simulink model "cosmic_ray_system_top"  (R2019a)
settings: Solver=VariableStepAuto  StartTime=0.0  StopTime=10.0  RelTol=1e-3
libraries: xbsIndex_r4 x3434, casper_library_misc x148, xps_library x3, casper_library_delays x1
(part 8 of 27)

== system cosmic_ray_system_top/Subsystem/wait_between_packets ==
  sim_1 : Inport
  convert1_1 : DataTypeConversion  OutDataTypeStr=fixdt('ufix32_En0')  LockScale=on
  convert2_1 : DataTypeConversion  OutDataTypeStr=fixdt('ufix32_En0')  ConvertRealWorld=Stored Integer (SI)  LockScale=on
  cosmic_ray_system_top_Subsystem_wait_between_packets_user_data_out : xbsIndex_r4/Gateway In  gui_display_data_type=Fixed-point  arith_type=Unsigned  n_bits=32  bin_pt=0  preci_type=Single  exp_width=8  frac_width=24  rows=1  columns=1  quantization="Round  (unbiased: +/- Inf)"  overflow=Saturate  period=1  UseAsADC=off  ADCChannel='1'  interface=None  automatic_assignment=on  address_offset=hex2dec('00')  intf_name=''  intf_description=''  default_value=0  timing_constraint=None  locs_specified=off  LOCs={}  io_standard={}  inherit_from_input=off  hdl_port=on  dbl_ovrd=off  block_type=gatewayin
  gain_1 : Gain
  io_delay : xbsIndex_r4/Delay  rst=off  infoeditControl=Selection of Reset will increase slice count due to use of real FFs and instead of SRLs  en=off  latency=0  reg_retiming=on  dbl_ovrd=off  block_type=delay
  reint1 : xbsIndex_r4/Reinterpret  force_arith_type=on  arith_type=Unsigned  force_bin_pt=on  bin_pt=0  block_type=reinterpret
  slice_reg : xbsIndex_r4/Slice  nbits=32  boolean_output=off  mode=Lower Bit Location + Width  bit1=0  base1=MSB of Input  bit0=0  base0=LSB of Input  dbl_ovrd=off  block_type=slice
  in_reg : Outport
  wires:
  cosmic_ray_system_top_Subsystem_wait_between_packets_user_data_out/1 -> io_delay/1
  sim_1/1 -> convert1_1/1
  convert1_1/1 -> convert2_1/1
  convert2_1/1 -> gain_1/1
  gain_1/1 -> cosmic_ray_system_top_Subsystem_wait_between_packets_user_data_out/1
  io_delay/1 -> slice_reg/1
  slice_reg/1 -> reint1/1
  reint1/1 -> in_reg/1

== system cosmic_ray_system_top/Subsystem/buffer_and_packetizer/bus_create ==
  in1 : Inport
  in2 : Inport  Port=2
  in3 : Inport  Port=3
  concatenate : xbsIndex_r4/Concat  num_inputs=3  dbl_ovrd=off  block_type=concat
  reinterpret1 : xbsIndex_r4/Reinterpret  force_arith_type=on  arith_type=Unsigned  force_bin_pt=on  bin_pt=0  block_type=reinterpret
      settings: infoedit="Changes signal type without altering the binary representation.   You can changed the signal between signed and unsigned, and relocate the binary point.<br><br>Hardware notes: In hardware this block costs nothing.<br><br>Example:  Suppose the input is 6 bits wide, signed, with 2 fractional bits, and the output is forced to unsigned with 0 fractional bits.  Then an input of -2.0 (1110.00 in binary 2's complement) becomes an output of 56 (111000 in binary)."
  reinterpret2 : xbsIndex_r4/Reinterpret  force_arith_type=on  arith_type=Unsigned  force_bin_pt=on  bin_pt=0  block_type=reinterpret
      settings: infoedit="Changes signal type without altering the binary representation.   You can changed the signal between signed and unsigned, and relocate the binary point.<br><br>Hardware notes: In hardware this block costs nothing.<br><br>Example:  Suppose the input is 6 bits wide, signed, with 2 fractional bits, and the output is forced to unsigned with 0 fractional bits.  Then an input of -2.0 (1110.00 in binary 2's complement) becomes an output of 56 (111000 in binary)."
  reinterpret3 : xbsIndex_r4/Reinterpret  force_arith_type=on  arith_type=Unsigned  force_bin_pt=on  bin_pt=0  block_type=reinterpret
  bus_out : Outport
  wires:
  concatenate/1 -> bus_out/1
  in1/1 -> reinterpret1/1
  reinterpret1/1 -> concatenate/1
  in2/1 -> reinterpret2/1
  reinterpret2/1 -> concatenate/2
  in3/1 -> reinterpret3/1
  reinterpret3/1 -> concatenate/3

== system cosmic_ray_system_top/Subsystem/buffer_and_packetizer/bus_create1 ==
  in1 : Inport
  in2 : Inport  Port=2
  in3 : Inport  Port=3
  concatenate : xbsIndex_r4/Concat  num_inputs=3  dbl_ovrd=off  block_type=concat
  reinterpret1 : xbsIndex_r4/Reinterpret  force_arith_type=on  arith_type=Unsigned  force_bin_pt=on  bin_pt=0  block_type=reinterpret
      settings: infoedit="Changes signal type without altering the binary representation.   You can changed the signal between signed and unsigned, and relocate the binary point.<br><br>Hardware notes: In hardware this block costs nothing.<br><br>Example:  Suppose the input is 6 bits wide, signed, with 2 fractional bits, and the output is forced to unsigned with 0 fractional bits.  Then an input of -2.0 (1110.00 in binary 2's complement) becomes an output of 56 (111000 in binary)."
  reinterpret2 : xbsIndex_r4/Reinterpret  force_arith_type=on  arith_type=Unsigned  force_bin_pt=on  bin_pt=0  block_type=reinterpret
      settings: infoedit="Changes signal type without altering the binary representation.   You can changed the signal between signed and unsigned, and relocate the binary point.<br><br>Hardware notes: In hardware this block costs nothing.<br><br>Example:  Suppose the input is 6 bits wide, signed, with 2 fractional bits, and the output is forced to unsigned with 0 fractional bits.  Then an input of -2.0 (1110.00 in binary 2's complement) becomes an output of 56 (111000 in binary)."
  reinterpret3 : xbsIndex_r4/Reinterpret  force_arith_type=on  arith_type=Unsigned  force_bin_pt=on  bin_pt=0  block_type=reinterpret
  bus_out : Outport
  wires:
  reinterpret3/1 -> concatenate/3
  in3/1 -> reinterpret3/1
  reinterpret2/1 -> concatenate/2
  in2/1 -> reinterpret2/1
  reinterpret1/1 -> concatenate/1
  in1/1 -> reinterpret1/1
  concatenate/1 -> bus_out/1

== system cosmic_ray_system_top/Subsystem/buffer_and_packetizer/bus_create2 ==
  in1 : Inport
  in2 : Inport  Port=2
  in3 : Inport  Port=3
  concatenate : xbsIndex_r4/Concat  num_inputs=3  dbl_ovrd=off  block_type=concat
  reinterpret1 : xbsIndex_r4/Reinterpret  force_arith_type=on  arith_type=Unsigned  force_bin_pt=on  bin_pt=0  block_type=reinterpret
      settings: infoedit="Changes signal type without altering the binary representation.   You can changed the signal between signed and unsigned, and relocate the binary point.<br><br>Hardware notes: In hardware this block costs nothing.<br><br>Example:  Suppose the input is 6 bits wide, signed, with 2 fractional bits, and the output is forced to unsigned with 0 fractional bits.  Then an input of -2.0 (1110.00 in binary 2's complement) becomes an output of 56 (111000 in binary)."
  reinterpret2 : xbsIndex_r4/Reinterpret  force_arith_type=on  arith_type=Unsigned  force_bin_pt=on  bin_pt=0  block_type=reinterpret
      settings: infoedit="Changes signal type without altering the binary representation.   You can changed the signal between signed and unsigned, and relocate the binary point.<br><br>Hardware notes: In hardware this block costs nothing.<br><br>Example:  Suppose the input is 6 bits wide, signed, with 2 fractional bits, and the output is forced to unsigned with 0 fractional bits.  Then an input of -2.0 (1110.00 in binary 2's complement) becomes an output of 56 (111000 in binary)."
  reinterpret3 : xbsIndex_r4/Reinterpret  force_arith_type=on  arith_type=Unsigned  force_bin_pt=on  bin_pt=0  block_type=reinterpret
  bus_out : Outport
  wires:
  concatenate/1 -> bus_out/1
  in1/1 -> reinterpret1/1
  reinterpret1/1 -> concatenate/1
  in2/1 -> reinterpret2/1
  reinterpret2/1 -> concatenate/2
  in3/1 -> reinterpret3/1
  reinterpret3/1 -> concatenate/3

== system cosmic_ray_system_top/Subsystem/buffer_and_packetizer/bus_create3 ==
  in1 : Inport
  in2 : Inport  Port=2
  in3 : Inport  Port=3
  concatenate : xbsIndex_r4/Concat  num_inputs=3  dbl_ovrd=off  block_type=concat
  reinterpret1 : xbsIndex_r4/Reinterpret  force_arith_type=on  arith_type=Unsigned  force_bin_pt=on  bin_pt=0  block_type=reinterpret
      settings: infoedit="Changes signal type without altering the binary representation.   You can changed the signal between signed and unsigned, and relocate the binary point.<br><br>Hardware notes: In hardware this block costs nothing.<br><br>Example:  Suppose the input is 6 bits wide, signed, with 2 fractional bits, and the output is forced to unsigned with 0 fractional bits.  Then an input of -2.0 (1110.00 in binary 2's complement) becomes an output of 56 (111000 in binary)."
  reinterpret2 : xbsIndex_r4/Reinterpret  force_arith_type=on  arith_type=Unsigned  force_bin_pt=on  bin_pt=0  block_type=reinterpret
      settings: infoedit="Changes signal type without altering the binary representation.   You can changed the signal between signed and unsigned, and relocate the binary point.<br><br>Hardware notes: In hardware this block costs nothing.<br><br>Example:  Suppose the input is 6 bits wide, signed, with 2 fractional bits, and the output is forced to unsigned with 0 fractional bits.  Then an input of -2.0 (1110.00 in binary 2's complement) becomes an output of 56 (111000 in binary)."
  reinterpret3 : xbsIndex_r4/Reinterpret  force_arith_type=on  arith_type=Unsigned  force_bin_pt=on  bin_pt=0  block_type=reinterpret
  bus_out : Outport
  wires:
  reinterpret3/1 -> concatenate/3
  in3/1 -> reinterpret3/1
  reinterpret2/1 -> concatenate/2
  in2/1 -> reinterpret2/1
  reinterpret1/1 -> concatenate/1
  in1/1 -> reinterpret1/1
  concatenate/1 -> bus_out/1

== system cosmic_ray_system_top/Subsystem/buffer_and_packetizer/bus_expand ==
  bus_in : Inport
  reinterpret{1..4} (4 alike) : xbsIndex_r4/Reinterpret  force_arith_type=on  arith_type=Unsigned  force_bin_pt=on  bin_pt=0  block_type=reinterpret
  slice1 : xbsIndex_r4/Slice  nbits=160  boolean_output=off  mode=Upper Bit Location + Width  bit1=-480  base1=MSB of Input  bit0=0  base0=LSB of Input  dbl_ovrd=off  block_type=slice
  slice2 : xbsIndex_r4/Slice  nbits=160  boolean_output=off  mode=Upper Bit Location + Width  bit1=-320  base1=MSB of Input  bit0=0  base0=LSB of Input  dbl_ovrd=off  block_type=slice
  slice3 : xbsIndex_r4/Slice  nbits=160  boolean_output=off  mode=Upper Bit Location + Width  bit1=-160  base1=MSB of Input  bit0=0  base0=LSB of Input  dbl_ovrd=off  block_type=slice
  slice4 : xbsIndex_r4/Slice  nbits=160  boolean_output=off  mode=Upper Bit Location + Width  bit1=0  base1=MSB of Input  bit0=0  base0=LSB of Input  dbl_ovrd=off  block_type=slice
  msb_out4 : Outport
  out3 : Outport  Port=2
  out2 : Outport  Port=3
  lsb_out1 : Outport  Port=4
  wires:
  bus_in/1 -> slice4/1, slice3/1, slice2/1, slice1/1
  slice4/1 -> reinterpret4/1
  reinterpret4/1 -> msb_out4/1
  slice3/1 -> reinterpret3/1
  reinterpret3/1 -> out3/1
  slice2/1 -> reinterpret2/1
  reinterpret2/1 -> out2/1
  slice1/1 -> reinterpret1/1
  reinterpret1/1 -> lsb_out1/1

== system cosmic_ray_system_top/Subsystem/buffer_and_packetizer/count-limited-counter ==
  en : Inport
  limit : Inport  Port=2
  Relational2 : xbsIndex_r4/Relational  mode=a>=b  op_type=Bool  en=off  latency=0  dbl_ovrd=off  block_type=relational
  word_counter1 : xbsIndex_r4/Counter  cnt_type=Free Running  cnt_to=257  operation=Up  start_count=0  cnt_by_val=1  arith_type=Unsigned  n_bits=32  bin_pt=0  load_pin=off  rst=on  en=on  explicit_period=on  period=1  use_behavioral_HDL=off  implementation=Fabric  dbl_ovrd=off  block_type=counter
  out : Outport
  wires:
  Relational2/1 -> word_counter1/1
  word_counter1/1 -> out/1, Relational2/1
  en/1 -> word_counter1/2
  limit/1 -> Relational2/2

== system cosmic_ray_system_top/Subsystem/buffer_and_packetizer/edge_detect11 ==
  in : Inport
  Delay : xbsIndex_r4/Delay  rst=off  infoeditControl=Selection of Reset will increase slice count due to use of real FFs and instead of SRLs  en=off  latency=1  reg_retiming=off  dbl_ovrd=off  block_type=delay
      settings: xl_area=[0, 0, 0, 0, 0, 0, 0]
  Inverter : xbsIndex_r4/Inverter  en=off  latency=0  dbl_ovrd=off  block_type=inv
      settings: xl_area=[0, 0, 0, 0, 0, 0, 0]
  edge_op : xbsIndex_r4/Logical  logical_function=AND  inputs=2  en=off  latency=0  precision=Full  arith_type=Unsigned  n_bits=8  bin_pt=2  align_bp=on  dbl_ovrd=off  block_type=logical
      settings: xl_area=[0, 0, 0, 0, 0, 0, 0]
  out : Outport
  wires:
  Delay/1 -> edge_op/2
  in/1 -> Delay/1, Inverter/1
  edge_op/1 -> out/1
  Inverter/1 -> edge_op/1

== system cosmic_ray_system_top/Subsystem/buffer_and_packetizer/edge_detect12 ==
  in : Inport
  Delay : xbsIndex_r4/Delay  rst=off  infoeditControl=Selection of Reset will increase slice count due to use of real FFs and instead of SRLs  en=off  latency=1  reg_retiming=off  dbl_ovrd=off  block_type=delay
      settings: xl_area=[0, 0, 0, 0, 0, 0, 0]
  Inverter : xbsIndex_r4/Inverter  en=off  latency=0  dbl_ovrd=off  block_type=inv
      settings: xl_area=[0, 0, 0, 0, 0, 0, 0]
  edge_op : xbsIndex_r4/Logical  logical_function=AND  inputs=2  en=off  latency=0  precision=Full  arith_type=Unsigned  n_bits=8  bin_pt=2  align_bp=on  dbl_ovrd=off  block_type=logical
      settings: xl_area=[0, 0, 0, 0, 0, 0, 0]
  out : Outport
  wires:
  Delay/1 -> edge_op/2
  in/1 -> Delay/1, Inverter/1
  edge_op/1 -> out/1
  Inverter/1 -> edge_op/1

== system cosmic_ray_system_top/Subsystem/buffer_and_packetizer/edge_detect13 ==
  in : Inport
  Delay : xbsIndex_r4/Delay  rst=off  infoeditControl=Selection of Reset will increase slice count due to use of real FFs and instead of SRLs  en=off  latency=1  reg_retiming=off  dbl_ovrd=off  block_type=delay
      settings: xl_area=[0, 0, 0, 0, 0, 0, 0]
  Inverter : xbsIndex_r4/Inverter  en=off  latency=0  dbl_ovrd=off  block_type=inv
      settings: xl_area=[0, 0, 0, 0, 0, 0, 0]
  edge_op : xbsIndex_r4/Logical  logical_function=AND  inputs=2  en=off  latency=0  precision=Full  arith_type=Unsigned  n_bits=8  bin_pt=2  align_bp=on  dbl_ovrd=off  block_type=logical
      settings: xl_area=[0, 0, 0, 0, 0, 0, 0]
  out : Outport
  wires:
  Inverter/1 -> edge_op/1
  edge_op/1 -> out/1
  in/1 -> Inverter/1, Delay/1
  Delay/1 -> edge_op/2

== system cosmic_ray_system_top/Subsystem/coincidence_trigger/bus_relational ==
  a : Inport
  b : Inport  Port=2
  misci : Inport  Port=3
  a_debus : Subsystem  AncestorBlock=casper_library_flow_control/bus_expand  mask(bus_expand){mode=divisions of arbitrary size, outputNum=1, outputWidth=[11  11  11  11  11  11  11  11  11  11  11  11  11  11  11  11  11  11  11  11  11  11  11  11  11  11  11  11  11  11  11  11  11  11  11  11  11  11  11  11  11  11  11  11  11  11  11  11  11  11  11  11  11  11  11  11  11  11  11  11  11  11  11  11], outputBinaryPt=[0  0  0  0  0  0  0  0  0  0  0  0  0  0  0  0  0  0  0  0  0  0  0  0  0  0  0  0  0  0  0  0  0  0  0  0  0  0  0  0  0  0  0  0  0  0  0  0  0  0  0  0  0  0  0  0  0  0  0  0  0  0  0  0], outputArithmeticType=[0  0  0  0  0  0  0  0  0  0  0  0  0  0  0  0  0  0  0  0  0  0  0  0  0  0  0  0  0  0  0  0  0  0  0  0  0  0  0  0  0  0  0  0  0  0  0  0  0  0  0  0  0  0  0  0  0  0  0  0  0  0  0  0], show_format=on, outputToWorkspace=off, variablePrefix=, outputToModelAsWell=on}
      mask prompts: outputNum "Number of outputs:"; outputWidth "Output width [msb ... lsb]:"; outputBinaryPt "Output binary point position [msb ... lsb]:"; outputArithmeticType "Output arithmetic type (ufix=0, fix=1, bool=2) [msb ... lsb]:"; show_format "Print format string?"; outputToWorkspace "Output to workspace?"; variablePrefix "Variable name prefix:"; outputToModelAsWell "Output to model as well?"
      mask help:
      | Expands a 'bus' made using a bus_create or Xilinx
      | concat block.
      | The input will be divided into the specified number
      | of outputs with the specified arithmetic types.
      | Divisions are made from most significant bit.
      mask init: same as cosmic_ray_system_top/Subsystem/buffer_and_packetizer/bus_expand
      settings: AttributesFormatString=64 outputs: uf11.0,uf11.0,uf11.0,uf11.0,uf11.0,uf11.0,uf11.0,uf11.0,uf11.0,uf11.0,uf11.0,uf11.0,uf11.0,uf11.0,uf11.0,uf11.0,uf11.0,uf11.0,uf11.0,uf11.0,uf11.0,uf11.0,uf11.0,uf11.0,uf11.0,uf11.0,uf11.0,uf11.0,uf11.0,uf11.0,uf11.0,uf11.0,uf11.0,uf11.0,uf11.0,uf11.0,uf11.0,uf11.0,uf11.0,uf11.0,uf11.0,uf11.0,uf11.0,uf11.0,uf11.0,uf11.0,uf11.0,uf11.0,uf11.0,uf11.0,uf11.0,uf11.0,uf11.0,uf11.0,uf11.0,uf11.0,uf11.0,uf11.0,uf11.0,uf11.0,uf11.0,uf11.0,uf11.0,uf11.0,
      mask TypeOptions mode: divisions of equal size | divisions of arbitrary size
      mask Callback mode: bus_expand_callback();
      mask Callback outputWidth: bus_expand_callback();
      mask Callback outputToWorkspace: bus_expand_callback();
  b_debus : Subsystem  AncestorBlock=casper_library_flow_control/bus_expand  mask(bus_expand){mode=divisions of arbitrary size, outputNum=1, outputWidth=[12], outputBinaryPt=[0], outputArithmeticType=[0], show_format=on, outputToWorkspace=off, variablePrefix=, outputToModelAsWell=on}
      mask prompts: outputNum "Number of outputs:"; outputWidth "Output width [msb ... lsb]:"; outputBinaryPt "Output binary point position [msb ... lsb]:"; outputArithmeticType "Output arithmetic type (ufix=0, fix=1, bool=2) [msb ... lsb]:"; show_format "Print format string?"; outputToWorkspace "Output to workspace?"; variablePrefix "Variable name prefix:"; outputToModelAsWell "Output to model as well?"
      mask help:
      | Expands a 'bus' made using a bus_create or Xilinx
      | concat block.
      | The input will be divided into the specified number
      | of outputs with the specified arithmetic types.
      | Divisions are made from most significant bit.
      mask init: same as cosmic_ray_system_top/Subsystem/buffer_and_packetizer/bus_expand
      settings: AttributesFormatString=1 outputs: uf12.0,
      mask TypeOptions mode: divisions of equal size | divisions of arbitrary size
      mask Callback mode: bus_expand_callback();
      mask Callback outputWidth: bus_expand_callback();
      mask Callback outputToWorkspace: bus_expand_callback();
  bussify : Subsystem  AncestorBlock=casper_library_flow_control/bus_create  mask(bus_create){inputNum=64}
      mask prompts: inputNum "Number of inputs:"
      mask init:
      | bus_create_init(gcb,...
      |     'inputNum', inputNum);
  dmisc : xbsIndex_r4/Delay  rst=off  infoeditControl=Selection of Reset will increase slice count due to use of real FFs and instead of SRLs  en=off  latency=1  reg_retiming=on  dbl_ovrd=off  block_type=delay
  relational{1..64} (64 alike) : xbsIndex_r4/Relational  mode=a>b  op_type=Bool  en=off  latency=1  dbl_ovrd=off  block_type=relational
  a>b : Outport
  misco : Outport  Port=2
  wires:
  a/1 -> a_debus/1(bus_in)
  b/1 -> b_debus/1(bus_in)
  a_debus/1(msb_out64) -> relational1/1
  b_debus/1(msb_lsb_out1) -> relational1/2, relational2/2, relational3/2, relational4/2, relational5/2, relational6/2, relational7/2, relational8/2, relational9/2, relational10/2, relational11/2, relational12/2, relational13/2, relational14/2, relational15/2, relational16/2, relational17/2, relational18/2, relational19/2, relational20/2, relational21/2, relational22/2, relational23/2, relational24/2, relational25/2, relational26/2, relational27/2, relational28/2, relational29/2, relational30/2, relational31/2, relational32/2, relational33/2, relational34/2, relational35/2, relational36/2, relational37/2, relational38/2, relational39/2, relational40/2, relational41/2, relational42/2, relational43/2, relational44/2, relational45/2, relational46/2, relational47/2, relational48/2, relational49/2, relational50/2, relational51/2, relational52/2, relational53/2, relational54/2, relational55/2, relational56/2, relational57/2, relational58/2, relational59/2, relational60/2, relational61/2, relational62/2, relational63/2, relational64/2
  a_debus/2(out63) -> relational2/1
  a_debus/3(out62) -> relational3/1
  a_debus/4(out61) -> relational4/1
  a_debus/5(out60) -> relational5/1
  a_debus/6(out59) -> relational6/1
  a_debus/7(out58) -> relational7/1
  a_debus/8(out57) -> relational8/1
  a_debus/9(out56) -> relational9/1
  a_debus/10(out55) -> relational10/1
  a_debus/11(out54) -> relational11/1
  a_debus/12(out53) -> relational12/1
  a_debus/13(out52) -> relational13/1
  a_debus/14(out51) -> relational14/1
  a_debus/15(out50) -> relational15/1
  a_debus/16(out49) -> relational16/1
  a_debus/17(out48) -> relational17/1
  a_debus/18(out47) -> relational18/1
  a_debus/19(out46) -> relational19/1
  a_debus/20(out45) -> relational20/1
  a_debus/21(out44) -> relational21/1
  a_debus/22(out43) -> relational22/1
  a_debus/23(out42) -> relational23/1
  a_debus/24(out41) -> relational24/1
  a_debus/25(out40) -> relational25/1
  a_debus/26(out39) -> relational26/1
  a_debus/27(out38) -> relational27/1
  a_debus/28(out37) -> relational28/1
  a_debus/29(out36) -> relational29/1
  a_debus/30(out35) -> relational30/1
  a_debus/31(out34) -> relational31/1
  a_debus/32(out33) -> relational32/1
  a_debus/33(out32) -> relational33/1
  a_debus/34(out31) -> relational34/1
  a_debus/35(out30) -> relational35/1
  a_debus/36(out29) -> relational36/1
  a_debus/37(out28) -> relational37/1
  a_debus/38(out27) -> relational38/1
  a_debus/39(out26) -> relational39/1
  a_debus/40(out25) -> relational40/1
  a_debus/41(out24) -> relational41/1
  a_debus/42(out23) -> relational42/1
  a_debus/43(out22) -> relational43/1
  a_debus/44(out21) -> relational44/1
  a_debus/45(out20) -> relational45/1
  a_debus/46(out19) -> relational46/1
  a_debus/47(out18) -> relational47/1
  a_debus/48(out17) -> relational48/1
  a_debus/49(out16) -> relational49/1
  a_debus/50(out15) -> relational50/1
  a_debus/51(out14) -> relational51/1
  a_debus/52(out13) -> relational52/1
  a_debus/53(out12) -> relational53/1
  a_debus/54(out11) -> relational54/1
  a_debus/55(out10) -> relational55/1
  a_debus/56(out9) -> relational56/1
  a_debus/57(out8) -> relational57/1
  a_debus/58(out7) -> relational58/1
  a_debus/59(out6) -> relational59/1
  a_debus/60(out5) -> relational60/1
  a_debus/61(out4) -> relational61/1
  a_debus/62(out3) -> relational62/1
  a_debus/63(out2) -> relational63/1
  a_debus/64(lsb_out1) -> relational64/1
  misci/1 -> dmisc/1
  relational1/1 -> bussify/1(in1)
  relational2/1 -> bussify/2(in2)
  relational3/1 -> bussify/3(in3)
  relational4/1 -> bussify/4(in4)
  relational5/1 -> bussify/5(in5)
  relational6/1 -> bussify/6(in6)
  relational7/1 -> bussify/7(in7)
  relational8/1 -> bussify/8(in8)
  relational9/1 -> bussify/9(in9)
  relational10/1 -> bussify/10(in10)
  relational11/1 -> bussify/11(in11)
  relational12/1 -> bussify/12(in12)
  relational13/1 -> bussify/13(in13)
  relational14/1 -> bussify/14(in14)
  relational15/1 -> bussify/15(in15)
  relational16/1 -> bussify/16(in16)
  relational17/1 -> bussify/17(in17)
  relational18/1 -> bussify/18(in18)
  relational19/1 -> bussify/19(in19)
  relational20/1 -> bussify/20(in20)
  relational21/1 -> bussify/21(in21)
  relational22/1 -> bussify/22(in22)
  relational23/1 -> bussify/23(in23)
  relational24/1 -> bussify/24(in24)
  relational25/1 -> bussify/25(in25)
  relational26/1 -> bussify/26(in26)
  relational27/1 -> bussify/27(in27)
  relational28/1 -> bussify/28(in28)
  relational29/1 -> bussify/29(in29)
  relational30/1 -> bussify/30(in30)
  relational31/1 -> bussify/31(in31)
  relational32/1 -> bussify/32(in32)
  relational33/1 -> bussify/33(in33)
  relational34/1 -> bussify/34(in34)
  relational35/1 -> bussify/35(in35)
  relational36/1 -> bussify/36(in36)
  relational37/1 -> bussify/37(in37)
  relational38/1 -> bussify/38(in38)
  relational39/1 -> bussify/39(in39)
  relational40/1 -> bussify/40(in40)
  relational41/1 -> bussify/41(in41)
  relational42/1 -> bussify/42(in42)
  relational43/1 -> bussify/43(in43)
  relational44/1 -> bussify/44(in44)
  relational45/1 -> bussify/45(in45)
  relational46/1 -> bussify/46(in46)
  relational47/1 -> bussify/47(in47)
  relational48/1 -> bussify/48(in48)
  relational49/1 -> bussify/49(in49)
  relational50/1 -> bussify/50(in50)
  relational51/1 -> bussify/51(in51)
  relational52/1 -> bussify/52(in52)
  relational53/1 -> bussify/53(in53)
  relational54/1 -> bussify/54(in54)
  relational55/1 -> bussify/55(in55)
  relational56/1 -> bussify/56(in56)
  relational57/1 -> bussify/57(in57)
  relational58/1 -> bussify/58(in58)
  relational59/1 -> bussify/59(in59)
  relational60/1 -> bussify/60(in60)
  relational61/1 -> bussify/61(in61)
  relational62/1 -> bussify/62(in62)
  relational63/1 -> bussify/63(in63)
  relational64/1 -> bussify/64(in64)
  bussify/1(bus_out) -> a>b/1
  dmisc/1 -> misco/1

== system cosmic_ray_system_top/Subsystem/coincidence_trigger/bus_relational1 ==
  a : Inport
  b : Inport  Port=2
  misci : Inport  Port=3
  a_debus : Subsystem  AncestorBlock=casper_library_flow_control/bus_expand  mask(bus_expand){mode=divisions of arbitrary size, outputNum=1, outputWidth=[11  11  11  11  11  11  11  11  11  11  11  11  11  11  11  11  11  11  11  11  11  11  11  11  11  11  11  11  11  11  11  11  11  11  11  11  11  11  11  11  11  11  11  11  11  11  11  11  11  11  11  11  11  11  11  11  11  11  11  11  11  11  11  11], outputBinaryPt=[0  0  0  0  0  0  0  0  0  0  0  0  0  0  0  0  0  0  0  0  0  0  0  0  0  0  0  0  0  0  0  0  0  0  0  0  0  0  0  0  0  0  0  0  0  0  0  0  0  0  0  0  0  0  0  0  0  0  0  0  0  0  0  0], outputArithmeticType=[0  0  0  0  0  0  0  0  0  0  0  0  0  0  0  0  0  0  0  0  0  0  0  0  0  0  0  0  0  0  0  0  0  0  0  0  0  0  0  0  0  0  0  0  0  0  0  0  0  0  0  0  0  0  0  0  0  0  0  0  0  0  0  0], show_format=on, outputToWorkspace=off, variablePrefix=, outputToModelAsWell=on}
      mask prompts: outputNum "Number of outputs:"; outputWidth "Output width [msb ... lsb]:"; outputBinaryPt "Output binary point position [msb ... lsb]:"; outputArithmeticType "Output arithmetic type (ufix=0, fix=1, bool=2) [msb ... lsb]:"; show_format "Print format string?"; outputToWorkspace "Output to workspace?"; variablePrefix "Variable name prefix:"; outputToModelAsWell "Output to model as well?"
      mask help:
      | Expands a 'bus' made using a bus_create or Xilinx
      | concat block.
      | The input will be divided into the specified number
      | of outputs with the specified arithmetic types.
      | Divisions are made from most significant bit.
      mask init: same as cosmic_ray_system_top/Subsystem/buffer_and_packetizer/bus_expand
      settings: AttributesFormatString=64 outputs: uf11.0,uf11.0,uf11.0,uf11.0,uf11.0,uf11.0,uf11.0,uf11.0,uf11.0,uf11.0,uf11.0,uf11.0,uf11.0,uf11.0,uf11.0,uf11.0,uf11.0,uf11.0,uf11.0,uf11.0,uf11.0,uf11.0,uf11.0,uf11.0,uf11.0,uf11.0,uf11.0,uf11.0,uf11.0,uf11.0,uf11.0,uf11.0,uf11.0,uf11.0,uf11.0,uf11.0,uf11.0,uf11.0,uf11.0,uf11.0,uf11.0,uf11.0,uf11.0,uf11.0,uf11.0,uf11.0,uf11.0,uf11.0,uf11.0,uf11.0,uf11.0,uf11.0,uf11.0,uf11.0,uf11.0,uf11.0,uf11.0,uf11.0,uf11.0,uf11.0,uf11.0,uf11.0,uf11.0,uf11.0,
      mask TypeOptions mode: divisions of equal size | divisions of arbitrary size
      mask Callback mode: bus_expand_callback();
      mask Callback outputWidth: bus_expand_callback();
      mask Callback outputToWorkspace: bus_expand_callback();
  b_debus : Subsystem  AncestorBlock=casper_library_flow_control/bus_expand  mask(bus_expand){mode=divisions of arbitrary size, outputNum=1, outputWidth=[12], outputBinaryPt=[0], outputArithmeticType=[0], show_format=on, outputToWorkspace=off, variablePrefix=, outputToModelAsWell=on}
      mask prompts: outputNum "Number of outputs:"; outputWidth "Output width [msb ... lsb]:"; outputBinaryPt "Output binary point position [msb ... lsb]:"; outputArithmeticType "Output arithmetic type (ufix=0, fix=1, bool=2) [msb ... lsb]:"; show_format "Print format string?"; outputToWorkspace "Output to workspace?"; variablePrefix "Variable name prefix:"; outputToModelAsWell "Output to model as well?"
      mask help:
      | Expands a 'bus' made using a bus_create or Xilinx
      | concat block.
      | The input will be divided into the specified number
      | of outputs with the specified arithmetic types.
      | Divisions are made from most significant bit.
      mask init: same as cosmic_ray_system_top/Subsystem/buffer_and_packetizer/bus_expand
      settings: AttributesFormatString=1 outputs: uf12.0,
      mask TypeOptions mode: divisions of equal size | divisions of arbitrary size
      mask Callback mode: bus_expand_callback();
      mask Callback outputWidth: bus_expand_callback();
      mask Callback outputToWorkspace: bus_expand_callback();
  bussify : Subsystem  AncestorBlock=casper_library_flow_control/bus_create  mask(bus_create){inputNum=64}
      mask prompts: inputNum "Number of inputs:"
      mask init:
      | bus_create_init(gcb,...
      |     'inputNum', inputNum);
  dmisc : xbsIndex_r4/Delay  rst=off  infoeditControl=Selection of Reset will increase slice count due to use of real FFs and instead of SRLs  en=off  latency=1  reg_retiming=on  dbl_ovrd=off  block_type=delay
  relational{1..64} (64 alike) : xbsIndex_r4/Relational  mode=a>b  op_type=Bool  en=off  latency=1  dbl_ovrd=off  block_type=relational
  a>b : Outport
  misco : Outport  Port=2
  wires:
  a/1 -> a_debus/1(bus_in)
  b/1 -> b_debus/1(bus_in)
  a_debus/1(msb_out64) -> relational1/1
  b_debus/1(msb_lsb_out1) -> relational1/2, relational2/2, relational3/2, relational4/2, relational5/2, relational6/2, relational7/2, relational8/2, relational9/2, relational10/2, relational11/2, relational12/2, relational13/2, relational14/2, relational15/2, relational16/2, relational17/2, relational18/2, relational19/2, relational20/2, relational21/2, relational22/2, relational23/2, relational24/2, relational25/2, relational26/2, relational27/2, relational28/2, relational29/2, relational30/2, relational31/2, relational32/2, relational33/2, relational34/2, relational35/2, relational36/2, relational37/2, relational38/2, relational39/2, relational40/2, relational41/2, relational42/2, relational43/2, relational44/2, relational45/2, relational46/2, relational47/2, relational48/2, relational49/2, relational50/2, relational51/2, relational52/2, relational53/2, relational54/2, relational55/2, relational56/2, relational57/2, relational58/2, relational59/2, relational60/2, relational61/2, relational62/2, relational63/2, relational64/2
  a_debus/2(out63) -> relational2/1
  a_debus/3(out62) -> relational3/1
  a_debus/4(out61) -> relational4/1
  a_debus/5(out60) -> relational5/1
  a_debus/6(out59) -> relational6/1
  a_debus/7(out58) -> relational7/1
  a_debus/8(out57) -> relational8/1
  a_debus/9(out56) -> relational9/1
  a_debus/10(out55) -> relational10/1
  a_debus/11(out54) -> relational11/1
  a_debus/12(out53) -> relational12/1
  a_debus/13(out52) -> relational13/1
  a_debus/14(out51) -> relational14/1
  a_debus/15(out50) -> relational15/1
  a_debus/16(out49) -> relational16/1
  a_debus/17(out48) -> relational17/1
  a_debus/18(out47) -> relational18/1
  a_debus/19(out46) -> relational19/1
  a_debus/20(out45) -> relational20/1
  a_debus/21(out44) -> relational21/1
  a_debus/22(out43) -> relational22/1
  a_debus/23(out42) -> relational23/1
  a_debus/24(out41) -> relational24/1
  a_debus/25(out40) -> relational25/1
  a_debus/26(out39) -> relational26/1
  a_debus/27(out38) -> relational27/1
  a_debus/28(out37) -> relational28/1
  a_debus/29(out36) -> relational29/1
  a_debus/30(out35) -> relational30/1
  a_debus/31(out34) -> relational31/1
  a_debus/32(out33) -> relational32/1
  a_debus/33(out32) -> relational33/1
  a_debus/34(out31) -> relational34/1
  a_debus/35(out30) -> relational35/1
  a_debus/36(out29) -> relational36/1
  a_debus/37(out28) -> relational37/1
  a_debus/38(out27) -> relational38/1
  a_debus/39(out26) -> relational39/1
  a_debus/40(out25) -> relational40/1
  a_debus/41(out24) -> relational41/1
  a_debus/42(out23) -> relational42/1
  a_debus/43(out22) -> relational43/1
  a_debus/44(out21) -> relational44/1
  a_debus/45(out20) -> relational45/1
  a_debus/46(out19) -> relational46/1
  a_debus/47(out18) -> relational47/1
  a_debus/48(out17) -> relational48/1
  a_debus/49(out16) -> relational49/1
  a_debus/50(out15) -> relational50/1
  a_debus/51(out14) -> relational51/1
  a_debus/52(out13) -> relational52/1
  a_debus/53(out12) -> relational53/1
  a_debus/54(out11) -> relational54/1
  a_debus/55(out10) -> relational55/1
  a_debus/56(out9) -> relational56/1
  a_debus/57(out8) -> relational57/1
  a_debus/58(out7) -> relational58/1
  a_debus/59(out6) -> relational59/1
  a_debus/60(out5) -> relational60/1
  a_debus/61(out4) -> relational61/1
  a_debus/62(out3) -> relational62/1
  a_debus/63(out2) -> relational63/1
  a_debus/64(lsb_out1) -> relational64/1
  misci/1 -> dmisc/1
  relational1/1 -> bussify/1(in1)
  relational2/1 -> bussify/2(in2)
  relational3/1 -> bussify/3(in3)
  relational4/1 -> bussify/4(in4)
  relational5/1 -> bussify/5(in5)
  relational6/1 -> bussify/6(in6)
  relational7/1 -> bussify/7(in7)
  relational8/1 -> bussify/8(in8)
  relational9/1 -> bussify/9(in9)
  relational10/1 -> bussify/10(in10)
  relational11/1 -> bussify/11(in11)
  relational12/1 -> bussify/12(in12)
  relational13/1 -> bussify/13(in13)
  relational14/1 -> bussify/14(in14)
  relational15/1 -> bussify/15(in15)
  relational16/1 -> bussify/16(in16)
  relational17/1 -> bussify/17(in17)
  relational18/1 -> bussify/18(in18)
  relational19/1 -> bussify/19(in19)
  relational20/1 -> bussify/20(in20)
  relational21/1 -> bussify/21(in21)
  relational22/1 -> bussify/22(in22)
  relational23/1 -> bussify/23(in23)
  relational24/1 -> bussify/24(in24)
  relational25/1 -> bussify/25(in25)
  relational26/1 -> bussify/26(in26)
  relational27/1 -> bussify/27(in27)
  relational28/1 -> bussify/28(in28)
  relational29/1 -> bussify/29(in29)
  relational30/1 -> bussify/30(in30)
  relational31/1 -> bussify/31(in31)
  relational32/1 -> bussify/32(in32)
  relational33/1 -> bussify/33(in33)
  relational34/1 -> bussify/34(in34)
  relational35/1 -> bussify/35(in35)
  relational36/1 -> bussify/36(in36)
  relational37/1 -> bussify/37(in37)
  relational38/1 -> bussify/38(in38)
  relational39/1 -> bussify/39(in39)
  relational40/1 -> bussify/40(in40)
  relational41/1 -> bussify/41(in41)
  relational42/1 -> bussify/42(in42)
  relational43/1 -> bussify/43(in43)
  relational44/1 -> bussify/44(in44)
  relational45/1 -> bussify/45(in45)
  relational46/1 -> bussify/46(in46)
  relational47/1 -> bussify/47(in47)
  relational48/1 -> bussify/48(in48)
  relational49/1 -> bussify/49(in49)
  relational50/1 -> bussify/50(in50)
  relational51/1 -> bussify/51(in51)
  relational52/1 -> bussify/52(in52)
  relational53/1 -> bussify/53(in53)
  relational54/1 -> bussify/54(in54)
  relational55/1 -> bussify/55(in55)
  relational56/1 -> bussify/56(in56)
  relational57/1 -> bussify/57(in57)
  relational58/1 -> bussify/58(in58)
  relational59/1 -> bussify/59(in59)
  relational60/1 -> bussify/60(in60)
  relational61/1 -> bussify/61(in61)
  relational62/1 -> bussify/62(in62)
  relational63/1 -> bussify/63(in63)
  relational64/1 -> bussify/64(in64)
  bussify/1(bus_out) -> a>b/1
  dmisc/1 -> misco/1

== system cosmic_ray_system_top/Subsystem/coincidence_trigger/custom_pulse_extend_with_sync ==
  note: Subtract one so that the actual length of the extended pulse is the input number of clock cycles.
  "in " : Inport
  "pulse_length " : Inport  Port=2
  sync_in : Inport  Port=3
  AddSub : xbsIndex_r4/AddSub  mode=Subtraction  use_carryin=off  use_carryout=off  en=off  latency=1  precision=Full  arith_type=Unsigned  n_bits=16  bin_pt=14  quantization=Truncate  overflow=Wrap  use_behavioral_HDL=off  hw_selection=Fabric  pipelined=off  dbl_ovrd=off  block_type=addsub
  Constant22 : xbsIndex_r4/Constant  const=1  gui_display_data_type=Fixed-point  arith_type=Unsigned  n_bits=12  bin_pt=0  preci_type=Single  exp_width=8  frac_width=24  explicit_period=on  period=1  equ=P=C  opselect=C  inp2=PCIN>>17  opr=+  inp1=P  carry=CIN  dbl_ovrd=off  block_type=constant
  Counter : xbsIndex_r4/Counter  cnt_type=Free Running  cnt_to=Inf  operation=Up  start_count=0  cnt_by_val=1  arith_type=Unsigned  n_bits=12  bin_pt=0  load_pin=off  rst=on  en=on  explicit_period=on  period=1  use_behavioral_HDL=off  implementation=Fabric  dbl_ovrd=off  block_type=counter
  Delay1 : xbsIndex_r4/Delay  rst=off  infoeditControl=Selection of Reset will increase slice count due to use of real FFs and instead of SRLs  en=off  latency=2  reg_retiming=on  dbl_ovrd=off  block_type=delay
  Relational : xbsIndex_r4/Relational  mode=a<b  op_type=Bool  en=off  latency=1  dbl_ovrd=off  block_type=relational
  Scope1 : Scope  Commented=on
  edge_detect : casper_library_misc/edge_detect  edge=Rising  polarity=Active High  x_in=[0 0.08 0.08 0.16 0.16 0.24 0.24 0.32 0.32 0.4]  y_in="[-1 -1  1  1  1  1  1  1  1  1]"  x_out=[0.6 0.68 0.68 0.76 0.76 0.84 0.84 0.92 0.92 1]  y_out="[-1 -1  1  1 -1 -1 -1 -1 -1 -1]"
  "out " : Outport
  sync_out : Outport  Port=2
  wires:
  AddSub/1 -> Relational/2
  Relational/1 -> Counter/2, "out "/1
  sync_in/1 -> Delay1/1
  "pulse_length "/1 -> AddSub/1
  Constant22/1 -> AddSub/2
  "in "/1 -> Scope1/1, edge_detect/1
  edge_detect/1 -> Counter/1
  Delay1/1 -> sync_out/1
  Counter/1 -> Relational/1

== system cosmic_ray_system_top/Subsystem/coincidence_trigger/custom_pulse_extend_with_sync1 ==
  note: Subtract one so that the actual length of the extended pulse is the input number of clock cycles.
  "in " : Inport
  "pulse_length " : Inport  Port=2
  sync_in : Inport  Port=3
  AddSub : xbsIndex_r4/AddSub  mode=Subtraction  use_carryin=off  use_carryout=off  en=off  latency=1  precision=Full  arith_type=Unsigned  n_bits=16  bin_pt=14  quantization=Truncate  overflow=Wrap  use_behavioral_HDL=off  hw_selection=Fabric  pipelined=off  dbl_ovrd=off  block_type=addsub
  Constant22 : xbsIndex_r4/Constant  const=1  gui_display_data_type=Fixed-point  arith_type=Unsigned  n_bits=12  bin_pt=0  preci_type=Single  exp_width=8  frac_width=24  explicit_period=on  period=1  equ=P=C  opselect=C  inp2=PCIN>>17  opr=+  inp1=P  carry=CIN  dbl_ovrd=off  block_type=constant
  Counter : xbsIndex_r4/Counter  cnt_type=Free Running  cnt_to=Inf  operation=Up  start_count=0  cnt_by_val=1  arith_type=Unsigned  n_bits=12  bin_pt=0  load_pin=off  rst=on  en=on  explicit_period=on  period=1  use_behavioral_HDL=off  implementation=Fabric  dbl_ovrd=off  block_type=counter
  Delay1 : xbsIndex_r4/Delay  rst=off  infoeditControl=Selection of Reset will increase slice count due to use of real FFs and instead of SRLs  en=off  latency=2  reg_retiming=on  dbl_ovrd=off  block_type=delay
  Relational : xbsIndex_r4/Relational  mode=a<b  op_type=Bool  en=off  latency=1  dbl_ovrd=off  block_type=relational
  Scope1 : Scope  Commented=on
  edge_detect : casper_library_misc/edge_detect  edge=Rising  polarity=Active High  x_in=[0 0.08 0.08 0.16 0.16 0.24 0.24 0.32 0.32 0.4]  y_in="[-1 -1  1  1  1  1  1  1  1  1]"  x_out=[0.6 0.68 0.68 0.76 0.76 0.84 0.84 0.92 0.92 1]  y_out="[-1 -1  1  1 -1 -1 -1 -1 -1 -1]"
  "out " : Outport
  sync_out : Outport  Port=2
  wires:
  Counter/1 -> Relational/1
  Delay1/1 -> sync_out/1
  edge_detect/1 -> Counter/1
  "in "/1 -> edge_detect/1, Scope1/1
  Constant22/1 -> AddSub/2
  "pulse_length "/1 -> AddSub/1
  sync_in/1 -> Delay1/1
  Relational/1 -> "out "/1, Counter/2
  AddSub/1 -> Relational/2

== system cosmic_ray_system_top/Subsystem/coincidence_trigger/square_bus_components ==
  IN : Inport
  sync_in : Inport  Port=2
  Absolute{,1..63} (64 alike) : xbsIndex_r4/Absolute  precision=Full  arith_type=Unsigned  n_bits=16  bin_pt=14  quantization=Truncate  overflow=Wrap  en=off  latency=1  dbl_ovrd=off  block_type=abs
  Delay7 : xbsIndex_r4/Delay  rst=off  infoeditControl=Selection of Reset will increase slice count due to use of real FFs and instead of SRLs  en=off  latency=1  reg_retiming=on  dbl_ovrd=off  block_type=delay
  Scope{,1..5} (6 alike) : Scope  Commented=on
  bus_create2 : Subsystem  AncestorBlock=casper_library_flow_control/bus_create  mask(bus_create){inputNum=64}
      mask prompts: inputNum "Number of inputs:"
      mask init:
      | bus_create_init(gcb,...
      |     'inputNum', inputNum);
  bus_expand : Subsystem  AncestorBlock=casper_library_flow_control/bus_expand  mask(bus_expand){mode=divisions of equal size, outputNum=64, outputWidth=10, outputBinaryPt=0, outputArithmeticType=0, show_format=off, outputToWorkspace=off, variablePrefix=out, outputToModelAsWell=on}
      mask prompts: outputNum "Number of outputs:"; outputWidth "Output width:"; outputBinaryPt "Output binary point position:"; outputArithmeticType "Output arithmetic type (ufix=0, fix=1, bool=2):"; show_format "Print format string?"; outputToWorkspace "Output to workspace?"; variablePrefix "Variable name prefix:"; outputToModelAsWell "Output to model as well?"
      mask help:
      | Expands a 'bus' made using a bus_create or Xilinx
      | concat block.
      | The input will be divided into the specified number
      | of outputs with the specified arithmetic types.
      | Divisions are made from most significant bit.
      mask init: same as cosmic_ray_system_top/Subsystem/buffer_and_packetizer/bus_expand
      settings: AttributesFormatString=64 outputs
      mask TypeOptions mode: divisions of equal size | divisions of arbitrary size
      mask Callback mode: bus_expand_callback();
      mask Callback outputWidth: bus_expand_callback();
      mask Callback outputToWorkspace: bus_expand_callback();
  OUT : Outport
  sync_out : Outport  Port=2
  wires:
  Delay7/1 -> sync_out/1
  sync_in/1 -> Delay7/1
  IN/1 -> bus_expand/1(bus_in)
  bus_create2/1(bus_out) -> OUT/1
  Absolute/1 -> bus_create2/1(in1)
  Absolute1/1 -> bus_create2/2(in2)
  Absolute2/1 -> bus_create2/3(in3)
  Absolute3/1 -> bus_create2/4(in4)
  Absolute4/1 -> bus_create2/5(in5)
  Absolute5/1 -> bus_create2/6(in6)
  Absolute6/1 -> bus_create2/7(in7)
  Absolute7/1 -> bus_create2/8(in8)
  Absolute8/1 -> bus_create2/9(in9)
  Absolute9/1 -> bus_create2/10(in10)
  Absolute10/1 -> bus_create2/11(in11)
  Absolute11/1 -> bus_create2/12(in12)
  Absolute12/1 -> bus_create2/13(in13)
  Absolute13/1 -> bus_create2/14(in14)
  Absolute14/1 -> bus_create2/15(in15)
  Absolute15/1 -> bus_create2/16(in16)
  Absolute16/1 -> bus_create2/17(in17)
  Absolute17/1 -> bus_create2/18(in18)
  Absolute24/1 -> bus_create2/19(in19)
  Absolute25/1 -> bus_create2/20(in20)
  Absolute26/1 -> bus_create2/21(in21)
  Absolute27/1 -> bus_create2/22(in22)
  Absolute28/1 -> bus_create2/23(in23)
  Absolute29/1 -> bus_create2/24(in24)
  Absolute30/1 -> bus_create2/25(in25)
  Absolute31/1 -> bus_create2/26(in26)
  Absolute18/1 -> bus_create2/27(in27)
  Absolute19/1 -> bus_create2/28(in28)
  Absolute20/1 -> bus_create2/29(in29)
  Absolute21/1 -> bus_create2/30(in30)
  Absolute22/1 -> bus_create2/31(in31)
  Absolute23/1 -> bus_create2/32(in32)
  Absolute32/1 -> bus_create2/33(in33)
  Absolute33/1 -> bus_create2/34(in34)
  Absolute44/1 -> bus_create2/35(in35)
  Absolute55/1 -> bus_create2/36(in36)
  Absolute58/1 -> bus_create2/37(in37)
  Absolute59/1 -> bus_create2/38(in38)
  Absolute60/1 -> bus_create2/39(in39)
  Absolute61/1 -> bus_create2/40(in40)
  Absolute62/1 -> bus_create2/41(in41)
  Absolute63/1 -> bus_create2/42(in42)
  Absolute34/1 -> bus_create2/43(in43)
  Absolute35/1 -> bus_create2/44(in44)
  Absolute36/1 -> bus_create2/45(in45)
  Absolute37/1 -> bus_create2/46(in46)
  Absolute38/1 -> bus_create2/47(in47)
  Absolute39/1 -> bus_create2/48(in48)
  Absolute40/1 -> bus_create2/49(in49)
  Absolute41/1 -> bus_create2/50(in50)
  Absolute49/1 -> bus_create2/51(in51)
  Absolute50/1 -> bus_create2/52(in52)
  Absolute51/1 -> bus_create2/53(in53)
  Absolute52/1 -> bus_create2/54(in54)
  Absolute53/1 -> bus_create2/55(in55)
  Absolute54/1 -> bus_create2/56(in56)
  Absolute56/1 -> bus_create2/57(in57)
  Absolute57/1 -> bus_create2/58(in58)
  Absolute42/1 -> bus_create2/59(in59)
  Absolute43/1 -> bus_create2/60(in60)
  Absolute45/1 -> bus_create2/61(in61)
  Absolute46/1 -> bus_create2/62(in62)
  Absolute47/1 -> bus_create2/63(in63)
  Absolute48/1 -> bus_create2/64(in64)
  bus_expand/1(msb_out64) -> Absolute/1
  bus_expand/2(out63) -> Absolute1/1
  bus_expand/3(out62) -> Absolute2/1
  bus_expand/4(out61) -> Absolute3/1
  bus_expand/5(out60) -> Absolute4/1
  bus_expand/6(out59) -> Absolute5/1
  bus_expand/7(out58) -> Absolute6/1
  bus_expand/8(out57) -> Absolute7/1
  bus_expand/9(out56) -> Absolute8/1
  bus_expand/10(out55) -> Absolute9/1
  bus_expand/11(out54) -> Absolute10/1
  bus_expand/12(out53) -> Absolute11/1
  bus_expand/13(out52) -> Absolute12/1
  bus_expand/14(out51) -> Absolute13/1
  bus_expand/15(out50) -> Absolute14/1
  bus_expand/16(out49) -> Absolute15/1
  bus_expand/17(out48) -> Absolute16/1
  bus_expand/18(out47) -> Absolute17/1
  bus_expand/19(out46) -> Absolute24/1
  bus_expand/20(out45) -> Absolute25/1
  bus_expand/21(out44) -> Absolute26/1
  bus_expand/22(out43) -> Absolute27/1
  bus_expand/23(out42) -> Absolute28/1
  bus_expand/24(out41) -> Absolute29/1
  bus_expand/25(out40) -> Absolute30/1
  bus_expand/26(out39) -> Absolute31/1
  bus_expand/27(out38) -> Absolute18/1
  bus_expand/28(out37) -> Absolute19/1
  bus_expand/29(out36) -> Absolute20/1
  bus_expand/30(out35) -> Absolute21/1
  bus_expand/31(out34) -> Absolute22/1
  bus_expand/32(out33) -> Absolute23/1
  bus_expand/33(out32) -> Absolute32/1
  bus_expand/34(out31) -> Absolute33/1
  bus_expand/35(out30) -> Absolute44/1
  bus_expand/36(out29) -> Absolute55/1
  bus_expand/37(out28) -> Absolute58/1
  bus_expand/38(out27) -> Absolute59/1
  bus_expand/39(out26) -> Absolute60/1
  bus_expand/40(out25) -> Absolute61/1
  bus_expand/41(out24) -> Absolute62/1
  bus_expand/42(out23) -> Absolute63/1
  bus_expand/43(out22) -> Absolute34/1
  bus_expand/44(out21) -> Absolute35/1
  bus_expand/45(out20) -> Absolute36/1
  bus_expand/46(out19) -> Absolute37/1
  bus_expand/47(out18) -> Absolute38/1
  bus_expand/48(out17) -> Absolute39/1
  bus_expand/49(out16) -> Absolute40/1
  bus_expand/50(out15) -> Absolute41/1
  bus_expand/51(out14) -> Absolute49/1
  bus_expand/52(out13) -> Absolute50/1
  bus_expand/53(out12) -> Absolute51/1
  bus_expand/54(out11) -> Absolute52/1
  bus_expand/55(out10) -> Absolute53/1
  bus_expand/56(out9) -> Absolute54/1
  bus_expand/57(out8) -> Absolute56/1
  bus_expand/58(out7) -> Absolute57/1
  bus_expand/59(out6) -> Absolute42/1
  bus_expand/60(out5) -> Absolute43/1
  bus_expand/61(out4) -> Absolute45/1
  bus_expand/62(out3) -> Absolute46/1
  bus_expand/63(out2) -> Absolute47/1
  bus_expand/64(lsb_out1) -> Absolute48/1
